simulink model "Cowley_321Lab3Sim"  (R2020b)
settings: Solver=VariableStepAuto  StartTime=0.0  StopTime=10.0  RelTol=1e-3
values from neighbouring files (symbols this model uses):
  d = 0    [Cowley_321Lab3.m]
  J = Jl + Jm    (= 2.029856e-05)    [Cowley_321Lab3.m]
  kb = 0.042    [Cowley_321Lab3.m]
  kt = 0.042    [Cowley_321Lab3.m]    (also in Cowley_321Project2.m = 190000)
  La = 0.0016    [Cowley_321Lab3.m]
  Ra = 8.4    [Cowley_321Lab3.m]
  vt = 3    [Cowley_321Lab3.m]
settings Model: Creator=mattcowley  LastModifiedBy=mattcowley
settings DataIOCC: SaveState=on

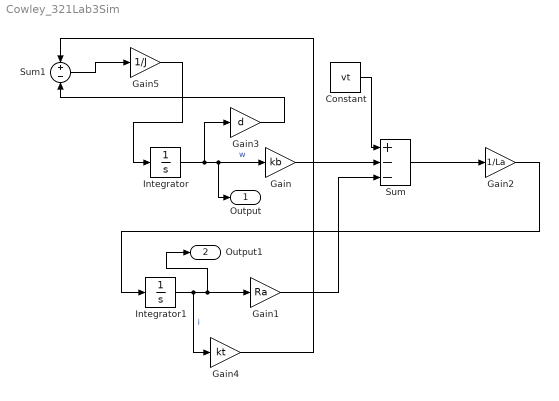
== system Cowley_321Lab3Sim ==
  Constant : Constant  Value=vt
  Gain : Gain  Gain=kb
  Gain1 : Gain  Gain=Ra
  Gain2 : Gain  Gain=1/La
  Gain3 : Gain  Gain=d
  Gain4 : Gain  Gain=kt
  Gain5 : Gain  Gain=1/J
  Integrator : Integrator
  Integrator1 : Integrator
  Sum : Sum  Inputs=+--
  Sum1 : Sum  Inputs=+-
  Output : Outport  SignalName=w
  Output1 : Outport  Port=2  SignalName=i
  wires:
  Integrator/1 -> Gain3/1, Output/1, Gain/1  "w"
  Constant/1 -> Sum/1
  Gain/1 -> Sum/2
  Integrator1/1 -> Gain4/1, Output1/1, Gain1/1  "i"
  Gain1/1 -> Sum/3
  Sum/1 -> Gain2/1
  Gain2/1 -> Integrator1/1
  Gain3/1 -> Sum1/2
  Gain4/1 -> Sum1/1
  Sum1/1 -> Gain5/1
  Gain5/1 -> Integrator/1
